simulink model "SrmAmLinearApcZhw3a"  (R2013b)
settings: Solver=ode45  StartTime=0.0  StopTime=10.0  MinStep=5e-5  RelTol=1e-3
InitFcn:
  | theta0=30*2*pi/360;
  | ks=2.44;
  | is=2;
  | lu=0.016;
  | rs=1.5
settings Model: Creator=mamingkai  LastModifiedBy=Think79

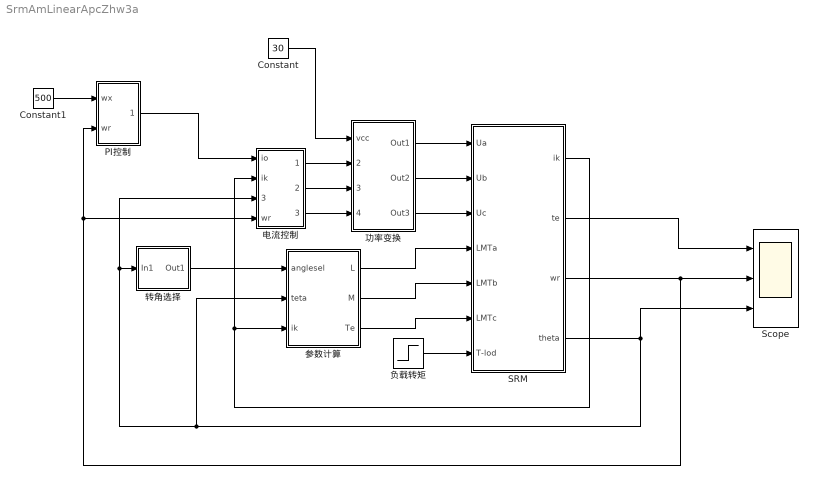
== system SrmAmLinearApcZhw3a ==
  Constant : Constant  Value=30
  Constant1 : Constant  Value=500
  PI控制 : Subsystem
  SRM : Subsystem
  Scope : Scope  NumInputPorts=3
      settings: YMin=-5~-5~-5  YMax=5~5~5
  功率变换 : Subsystem
  参数计算 : Subsystem
  电流控制 : Subsystem
  负载转矩 : Step  SampleTime=0
  转角选择 : Subsystem
  wires:
  Constant1/1 -> PI控制/1(wx)
  电流控制/1(Out1) -> 功率变换/2(PUSEA)
  电流控制/2(Out2) -> 功率变换/3(PUDEB)
  电流控制/3(Out3) -> 功率变换/4(PUSEC)
  PI控制/1(Out1) -> 电流控制/1(io)
  Constant/1 -> 功率变换/1(vcc)
  功率变换/1(Out1) -> SRM/1(Ua)
  功率变换/2(Out2) -> SRM/2(Ub)
  功率变换/3(Out3) -> SRM/3(Uc)
  转角选择/1(Out1) -> 参数计算/1("anglesel ")
  SRM/1(ik) -> 电流控制/2(ik), 参数计算/3(ik)
  SRM/3(wr) -> PI控制/2(wr), 电流控制/4(wr), Scope/2
  SRM/4(theta) -> Scope/3, 参数计算/2(teta), 电流控制/3(teta), 转角选择/1(In1)
  SRM/2(te) -> Scope/1
  参数计算/1(L) -> SRM/4(LMTa)
  参数计算/2(M) -> SRM/5(LMTb)
  参数计算/3(Te) -> SRM/6(LMTc)
  负载转矩/1 -> SRM/7(T-lod)

== system SrmAmLinearApcZhw3a/PI控制 ==
  wx : Inport
  wr : Inport  Port=2
  Gain : Gain
  Gain1 : Gain
  Integrator : Integrator
  Saturation : Saturate
  netsum : Sum  Inputs=2  SaturateOnIntegerOverflow=on  InputSameDT=on  OutDataTypeStr=Inherit: Same as first input
  netsum1 : Sum  Inputs=+-  SaturateOnIntegerOverflow=on  InputSameDT=on  OutDataTypeStr=Inherit: Same as first input
  Out1 : Outport
  wires:
  wx/1 -> netsum1/1
  wr/1 -> netsum1/2
  netsum1/1 -> Gain/1, Gain1/1
  Gain1/1 -> Integrator/1
  Integrator/1 -> netsum/2
  Gain/1 -> netsum/1
  netsum/1 -> Saturation/1
  Saturation/1 -> Out1/1

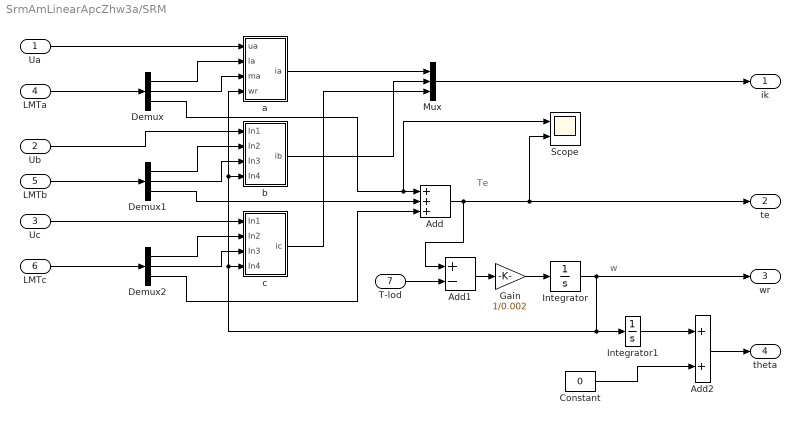
== system SrmAmLinearApcZhw3a/SRM ==
  note: w
  note: Te
  Ua : Inport
  Ub : Inport  Port=2
  Uc : Inport  Port=3
  LMTa : Inport  Port=4
  LMTb : Inport  Port=5
  LMTc : Inport  Port=6
  T-lod : Inport  Port=7
  Add : Sum  Inputs=+++
  Add1 : Sum  Inputs=+-
  Add2 : Sum
  Constant : Constant  Value=0
  Demux : Demux  Outputs=3
  Demux1 : Demux  Outputs=3
  Demux2 : Demux  Outputs=3
  Gain : Gain  Gain=1/0.002
  Integrator : Integrator
  Integrator1 : Integrator
  Mux : Mux  Inputs=3
  Scope : Scope  NumInputPorts=2
      settings: YMin=-5~-5  YMax=5~5
  a : Subsystem
  b : Subsystem
  c : Subsystem
  ik : Outport
  te : Outport  Port=2
  wr : Outport  Port=3
  theta : Outport  Port=4
  wires:
  LMTa/1 -> Demux/1
  Demux/1 -> a/2(la)
  Demux/2 -> a/3(ma)
  Demux/3 -> Scope/1, Add/1
  Ub/1 -> b/1(In1)
  Demux1/1 -> b/2(In2)
  Demux1/2 -> b/3(In3)
  Demux1/3 -> Add/2
  Uc/1 -> c/1(In1)
  LMTc/1 -> Demux2/1
  LMTb/1 -> Demux1/1
  Demux2/1 -> c/2(In2)
  Demux2/2 -> c/3(In3)
  Demux2/3 -> Add/3
  Integrator/1 -> wr/1, c/4(In4), b/4(In4), a/4(wr), Integrator1/1
  a/1(ia) -> Mux/1
  b/1("ib ") -> Mux/2
  c/1(ic) -> Mux/3
  Mux/1 -> ik/1
  Add/1 -> te/1, Scope/2, Add1/1
  T-lod/1 -> Add1/2
  Add1/1 -> Gain/1
  Gain/1 -> Integrator/1
  Add2/1 -> theta/1
  Integrator1/1 -> Add2/1
  Constant/1 -> Add2/2
  Ua/1 -> a/1(ua)

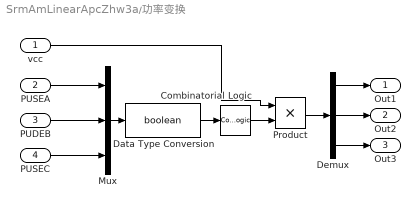
== system SrmAmLinearApcZhw3a/功率变换 ==
  vcc : Inport
  PUSEA : Inport  Port=2
  PUDEB : Inport  Port=3
  PUSEC : Inport  Port=4
  Combinatorial Logic : CombinatorialLogic  TruthTable=[0 0 0 ;0 0 1;0 1 0;0 1 1;1 0 0;1 0 1;1 1 0;1 1 1]
  Data Type Conversion : DataTypeConversion  OutDataTypeStr=boolean
  Demux : Demux  Outputs=3
  Mux : Mux  Inputs=3
  Product : Product
  Out1 : Outport
  Out2 : Outport  Port=2
  Out3 : Outport  Port=3
  wires:
  PUSEA/1 -> Mux/1
  Demux/1 -> Out1/1
  Product/1 -> Demux/1
  Demux/2 -> Out2/1
  Demux/3 -> Out3/1
  PUDEB/1 -> Mux/2
  PUSEC/1 -> Mux/3
  Combinatorial Logic/1 -> Product/2
  vcc/1 -> Product/1
  Mux/1 -> Data Type Conversion/1
  Data Type Conversion/1 -> Combinatorial Logic/1

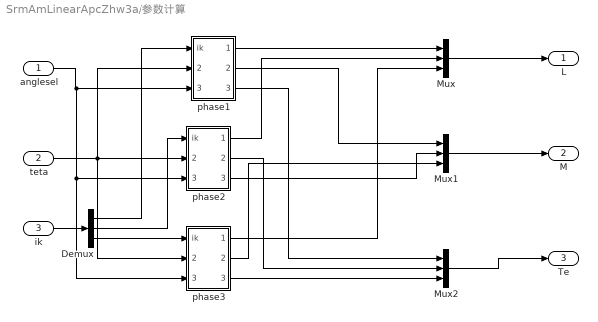
== system SrmAmLinearApcZhw3a/参数计算 ==
  "anglesel " : Inport
  teta : Inport  Port=2
  ik : Inport  Port=3
  Demux : Demux  Outputs=3
  Mux : Mux  Inputs=3
  Mux1 : Mux  Inputs=3
  Mux2 : Mux  Inputs=3
  phase1 : Subsystem
  phase2 : Subsystem
  phase3 : Subsystem
  L : Outport
  M : Outport  Port=2
  Te : Outport  Port=3
  wires:
  teta/1 -> phase3/2(theta), phase2/2(theta), phase1/2(theta)
  Mux/1 -> L/1
  "anglesel "/1 -> phase3/3(angle), phase2/3(angle), phase1/3(angle)
  ik/1 -> Demux/1
  Demux/1 -> phase1/1(ik)
  Demux/2 -> phase2/1(ik)
  Demux/3 -> phase3/1(ik)
  phase1/1(Out1) -> Mux/1
  phase1/2(Out2) -> Mux1/1
  phase1/3(Out3) -> Mux2/1
  phase2/1(Out1) -> Mux/2
  phase2/3(Out3) -> Mux1/2
  phase2/2(Out2) -> Mux2/2
  phase3/1(Out1) -> Mux/3
  phase3/2(Out2) -> Mux1/3
  phase3/3(Out3) -> Mux2/3
  Mux1/1 -> M/1
  Mux2/1 -> Te/1

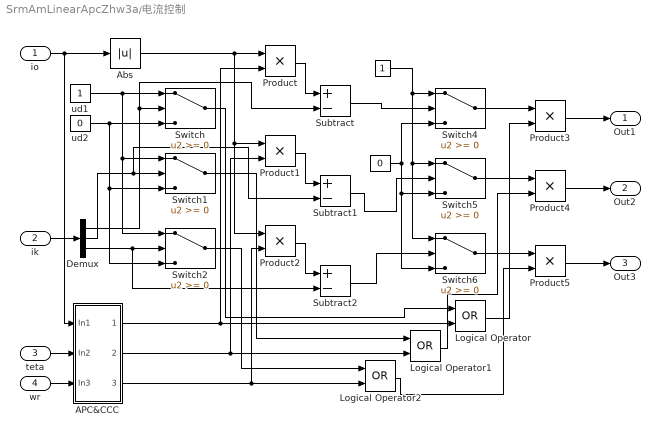
== system SrmAmLinearApcZhw3a/电流控制 ==
  io : Inport
  ik : Inport  Port=2
  teta : Inport  Port=3
  wr : Inport  Port=4
  " " : Constant
  " " : Constant  Value=0
  APC&CCC : Subsystem
  Abs : Abs
  Demux : Demux  Outputs=3
  Logical Operator : Logic  Operator=OR  AllPortsSameDT=off  OutDataTypeStr=boolean
  Logical Operator1 : Logic  Operator=OR  AllPortsSameDT=off  OutDataTypeStr=boolean
  Logical Operator2 : Logic  Operator=OR  AllPortsSameDT=off  OutDataTypeStr=boolean
  Product{,1..5} (6 alike) : Product
  Subtract : Sum  Inputs=+-
  Subtract1 : Sum  Inputs=+-
  Subtract2 : Sum  Inputs=+-
  Switch{,1..2,4..6} (6 alike) : Switch
  ud1 : Constant
  ud2 : Constant  Value=0
  Out1 : Outport
  Out2 : Outport  Port=2
  Out3 : Outport  Port=3
  wires:
  ik/1 -> Demux/1
  io/1 -> APC&CCC/1(In1), Abs/1
  Abs/1 -> Product2/1, Product1/1, Product/1
  ud1/1 -> Switch2/1, Switch1/1, Switch/1
  ud2/1 -> Switch2/3, Switch1/3, Switch/3
  teta/1 -> APC&CCC/2(In2)
  Demux/1 -> Subtract/2, Switch/2
  Demux/3 -> Subtract2/2, Switch2/2
  Demux/2 -> Subtract1/2, Switch1/2
  APC&CCC/1(Out1) -> Product/2, Logical Operator/2
  APC&CCC/2(Out2) -> Product1/2, Logical Operator1/2
  APC&CCC/3(Out3) -> Product2/2, Logical Operator2/2
  Switch/1 -> Logical Operator/1
  Switch1/1 -> Logical Operator1/1
  Switch2/1 -> Logical Operator2/1
  Product/1 -> Subtract/1
  Product1/1 -> Subtract1/1
  Product2/1 -> Subtract2/1
  " "/1 -> Switch6/1, Switch5/1, Switch4/1
  " "/1 -> Switch6/3, Switch5/3, Switch4/3
  wr/1 -> APC&CCC/3(In3)
  Logical Operator/1 -> Product3/2
  Logical Operator1/1 -> Product4/2
  Logical Operator2/1 -> Product5/2
  Switch6/1 -> Product5/1
  Switch5/1 -> Product4/1
  Switch4/1 -> Product3/1
  Product3/1 -> Out1/1
  Product4/1 -> Out2/1
  Product5/1 -> Out3/1
  Subtract1/1 -> Switch5/2
  Subtract/1 -> Switch4/2
  Subtract2/1 -> Switch6/2

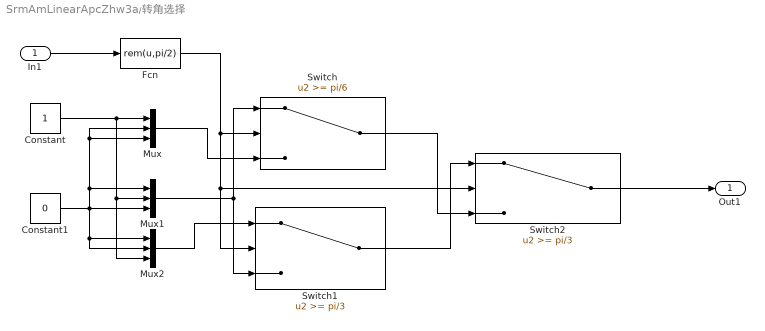
== system SrmAmLinearApcZhw3a/转角选择 ==
  In1 : Inport
  Constant : Constant
  Constant1 : Constant  Value=0
  Fcn : Fcn  Expr=rem(u,pi/2)
  Mux : Mux  Inputs=3
  Mux1 : Mux  Inputs=3
  Mux2 : Mux  Inputs=3
  Switch : Switch  Threshold=pi/6
  Switch1 : Switch  Threshold=pi/3
  Switch2 : Switch  Threshold=pi/3
  Out1 : Outport
  wires:
  In1/1 -> Fcn/1
  Constant/1 -> Mux2/3, Mux1/2, Mux/1
  Mux/1 -> Switch/3
  Constant1/1 -> Mux/3, Mux/2, Mux1/1, Mux2/2, Mux2/1, Mux1/3
  Mux1/1 -> Switch1/3, Switch/1
  Mux2/1 -> Switch1/1
  Fcn/1 -> Switch2/2, Switch1/2, Switch/2
  Switch/1 -> Switch2/3
  Switch1/1 -> Switch2/1
  Switch2/1 -> Out1/1

== system SrmAmLinearApcZhw3a/SRM/a ==
  ua : Inport
  la : Inport  Port=2
  ma : Inport  Port=3
  wr : Inport  Port=4
  Add : Sum  Inputs=+--
  Fcn : Fcn  Expr=1/u
  Gain : Gain  Gain=rs
  Integrator : Integrator
  Product : Product
  Product1 : Product
  ia : Outport
  wires:
  wr/1 -> Product/2
  Integrator/1 -> Gain/1, ia/1
  ma/1 -> Product/1
  la/1 -> Fcn/1
  ua/1 -> Add/1
  Gain/1 -> Add/2
  Product/1 -> Add/3
  Add/1 -> Product1/1
  Fcn/1 -> Product1/2
  Product1/1 -> Integrator/1

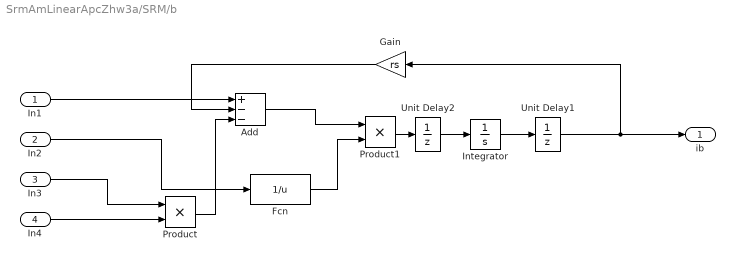
== system SrmAmLinearApcZhw3a/SRM/b ==
  In1 : Inport
  In2 : Inport  Port=2
  In3 : Inport  Port=3
  In4 : Inport  Port=4
  Add : Sum  Inputs=+--
  Fcn : Fcn  Expr=1/u
  Gain : Gain  Gain=rs
  Integrator : Integrator
  Product : Product
  Product1 : Product
  Unit Delay1 : UnitDelay  SampleTime=-1
  Unit Delay2 : UnitDelay  SampleTime=-1
  "ib " : Outport
  wires:
  In4/1 -> Product/2
  Integrator/1 -> Unit Delay1/1
  In3/1 -> Product/1
  In2/1 -> Fcn/1
  In1/1 -> Add/1
  Gain/1 -> Add/2
  Product/1 -> Add/3
  Add/1 -> Product1/1
  Fcn/1 -> Product1/2
  Product1/1 -> Unit Delay2/1
  Unit Delay2/1 -> Integrator/1
  Unit Delay1/1 -> Gain/1, "ib "/1

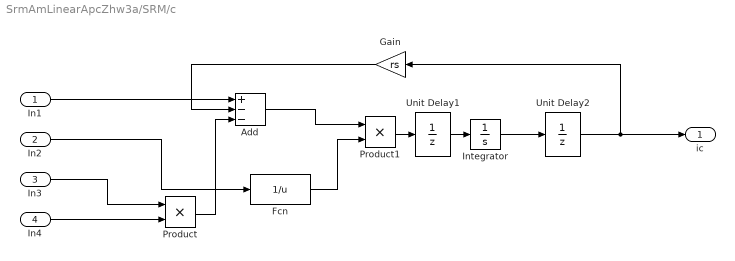
== system SrmAmLinearApcZhw3a/SRM/c ==
  In1 : Inport
  In2 : Inport  Port=2
  In3 : Inport  Port=3
  In4 : Inport  Port=4
  Add : Sum  Inputs=+--
  Fcn : Fcn  Expr=1/u
  Gain : Gain  Gain=rs
  Integrator : Integrator  InitialCondition=1e-5
  Product : Product
  Product1 : Product
  Unit Delay1 : UnitDelay  SampleTime=-1
  Unit Delay2 : UnitDelay  SampleTime=-1
  ic : Outport
  wires:
  In4/1 -> Product/2
  Integrator/1 -> Unit Delay2/1
  In3/1 -> Product/1
  In2/1 -> Fcn/1
  In1/1 -> Add/1
  Gain/1 -> Add/2
  Product/1 -> Add/3
  Add/1 -> Product1/1
  Fcn/1 -> Product1/2
  Product1/1 -> Unit Delay1/1
  Unit Delay2/1 -> Gain/1, ic/1
  Unit Delay1/1 -> Integrator/1

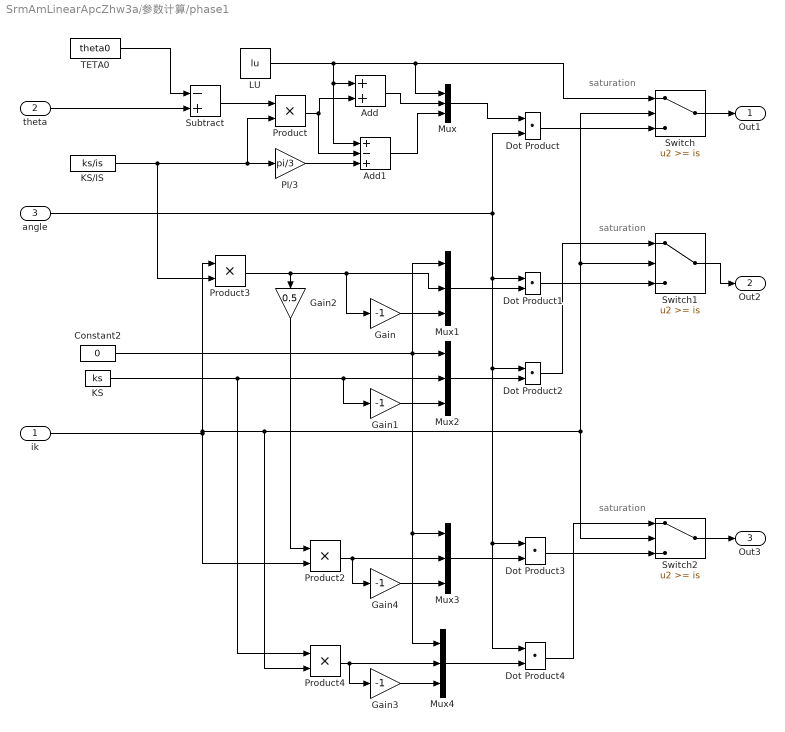
== system SrmAmLinearApcZhw3a/参数计算/phase1 ==
  note: saturation
  note: saturation
  note: saturation
  ik : Inport
  theta : Inport  Port=2
  angle : Inport  Port=3
  Add : Sum
  Add1 : Sum  Inputs=+-+
  Constant2 : Constant  Value=0
  Dot Product{,1..4} (5 alike) : DotProduct  InputSameDT=on  OutDataTypeStr=Inherit: Inherit via internal rule
  Gain{,1,3..4} (4 alike) : Gain  Gain=-1
  Gain2 : Gain  Gain=0.5
  KS : Constant  Value=ks
  KS/IS : Constant  Value=ks/is
  LU : Constant  Value=lu
  Mux{,1..4} (5 alike) : Mux  Inputs=3
  PI/3 : Gain  Gain=pi/3
  Product{,2..4} (4 alike) : Product
  Subtract : Sum  Inputs=-+
  Switch : Switch  Threshold=is
  Switch1 : Switch  Threshold=is
  Switch2 : Switch  Threshold=is
  TETA0 : Constant  Value=theta0
  Out1 : Outport
  Out2 : Outport  Port=2
  Out3 : Outport  Port=3
  wires:
  Switch/1 -> Out1/1
  theta/1 -> Subtract/2
  TETA0/1 -> Subtract/1
  Subtract/1 -> Product/1
  KS/IS/1 -> Product3/2, PI/3/1, Product/2
  LU/1 -> Switch/1, Mux/1, Add1/1, Add/1
  Product/1 -> Add1/2, Add/2
  PI/3/1 -> Add1/3
  Add/1 -> Mux/2
  Add1/1 -> Mux/3
  Mux/1 -> Dot Product/1
  Dot Product/1 -> Switch/3
  ik/1 -> Product3/1, Product4/2, Switch/2, Switch1/2, Switch2/2, Product2/2
  angle/1 -> Dot Product4/1, Dot Product3/1, Dot Product2/1, Dot Product1/1, Dot Product/2
  Mux4/1 -> Dot Product4/2
  Constant2/1 -> Mux1/1, Mux4/1, Mux3/1, Mux2/1
  Mux3/1 -> Dot Product3/2
  Mux2/1 -> Dot Product2/2
  Mux1/1 -> Dot Product1/2
  KS/1 -> Product4/1, Gain1/1, Mux2/2
  Product3/1 -> Gain/1, Mux1/2, Gain2/1
  Gain/1 -> Mux1/3
  Gain2/1 -> Product2/1
  Product4/1 -> Mux4/2, Gain3/1
  Gain3/1 -> Mux4/3
  Dot Product4/1 -> Switch2/1
  Dot Product3/1 -> Switch2/3
  Dot Product2/1 -> Switch1/1
  Dot Product1/1 -> Switch1/3
  Switch1/1 -> Out2/1
  Switch2/1 -> Out3/1
  Product2/1 -> Gain4/1, Mux3/2
  Gain4/1 -> Mux3/3
  Gain1/1 -> Mux2/3

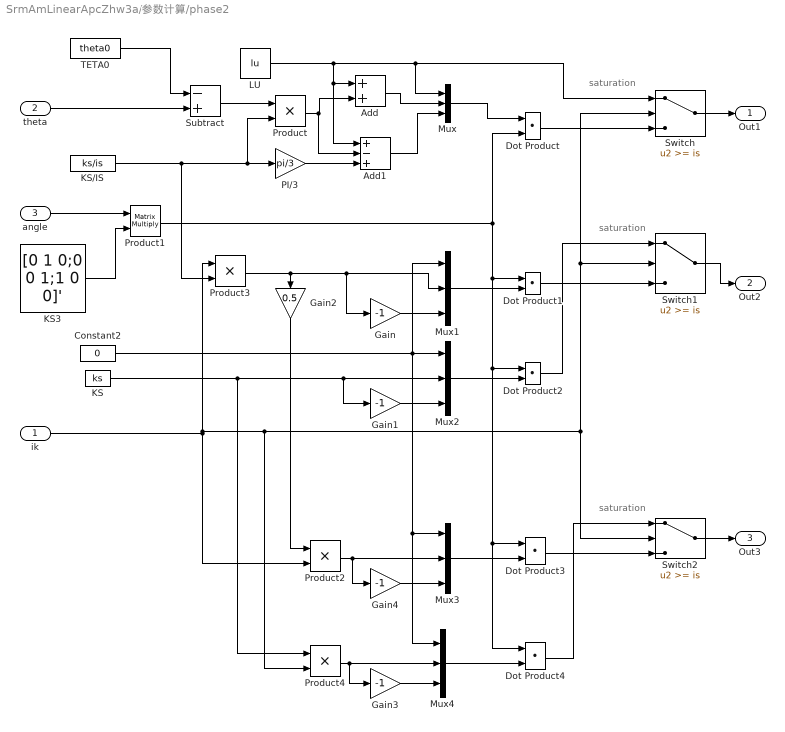
== system SrmAmLinearApcZhw3a/参数计算/phase2 ==
  note: saturation
  note: saturation
  note: saturation
  ik : Inport
  theta : Inport  Port=2
  angle : Inport  Port=3
  Add : Sum
  Add1 : Sum  Inputs=+-+
  Constant2 : Constant  Value=0
  Dot Product{,1..4} (5 alike) : DotProduct  InputSameDT=on  OutDataTypeStr=Inherit: Inherit via internal rule
  Gain{,1,3..4} (4 alike) : Gain  Gain=-1
  Gain2 : Gain  Gain=0.5
  KS : Constant  Value=ks
  KS/IS : Constant  Value=ks/is
  KS3 : Constant  Value="[0 1 0;0  0 1;1 0 0]'"  VectorParams1D=off
  LU : Constant  Value=lu
  Mux{,1..4} (5 alike) : Mux  Inputs=3
  PI/3 : Gain  Gain=pi/3
  Product{,2..4} (4 alike) : Product
  Product1 : Product  Multiplication=Matrix(*)
  Subtract : Sum  Inputs=-+
  Switch : Switch  Threshold=is
  Switch1 : Switch  Threshold=is
  Switch2 : Switch  Threshold=is
  TETA0 : Constant  Value=theta0
  Out1 : Outport
  Out2 : Outport  Port=2
  Out3 : Outport  Port=3
  wires:
  Switch/1 -> Out1/1
  theta/1 -> Subtract/2
  TETA0/1 -> Subtract/1
  Subtract/1 -> Product/1
  KS/IS/1 -> Product3/2, PI/3/1, Product/2
  LU/1 -> Switch/1, Mux/1, Add1/1, Add/1
  Product/1 -> Add1/2, Add/2
  PI/3/1 -> Add1/3
  Add/1 -> Mux/2
  Add1/1 -> Mux/3
  Mux/1 -> Dot Product/1
  Dot Product/1 -> Switch/3
  ik/1 -> Product3/1, Product4/2, Switch/2, Switch1/2, Switch2/2, Product2/2
  Product1/1 -> Dot Product/2, Dot Product4/1, Dot Product3/1, Dot Product2/1, Dot Product1/1
  Mux4/1 -> Dot Product4/2
  Constant2/1 -> Mux1/1, Mux4/1, Mux3/1, Mux2/1
  Mux3/1 -> Dot Product3/2
  Mux2/1 -> Dot Product2/2
  Mux1/1 -> Dot Product1/2
  KS/1 -> Product4/1, Gain1/1, Mux2/2
  Product3/1 -> Gain/1, Mux1/2, Gain2/1
  Gain/1 -> Mux1/3
  Gain2/1 -> Product2/1
  Product4/1 -> Mux4/2, Gain3/1
  Gain3/1 -> Mux4/3
  Dot Product4/1 -> Switch2/1
  Dot Product3/1 -> Switch2/3
  Dot Product2/1 -> Switch1/1
  Dot Product1/1 -> Switch1/3
  Switch1/1 -> Out2/1
  Switch2/1 -> Out3/1
  Product2/1 -> Gain4/1, Mux3/2
  Gain4/1 -> Mux3/3
  Gain1/1 -> Mux2/3
  KS3/1 -> Product1/2
  angle/1 -> Product1/1

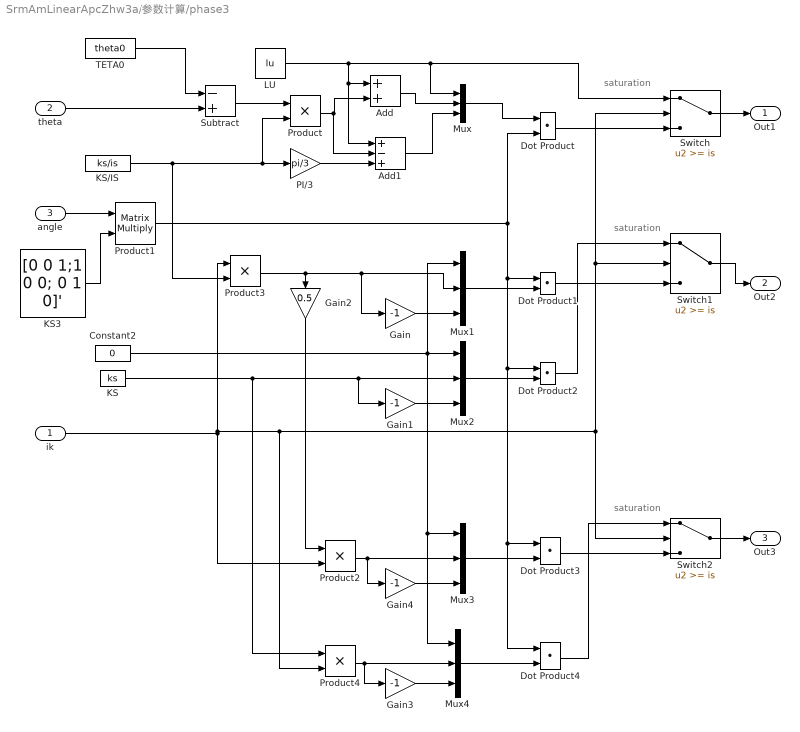
== system SrmAmLinearApcZhw3a/参数计算/phase3 ==
  note: saturation
  note: saturation
  note: saturation
  ik : Inport
  theta : Inport  Port=2
  angle : Inport  Port=3
  Add : Sum
  Add1 : Sum  Inputs=+-+
  Constant2 : Constant  Value=0
  Dot Product{,1..4} (5 alike) : DotProduct  InputSameDT=on  OutDataTypeStr=Inherit: Inherit via internal rule
  Gain{,1,3..4} (4 alike) : Gain  Gain=-1
  Gain2 : Gain  Gain=0.5
  KS : Constant  Value=ks
  KS/IS : Constant  Value=ks/is
  KS3 : Constant  Value="[0 0 1;1 0  0; 0 1 0]'"  VectorParams1D=off
  LU : Constant  Value=lu
  Mux{,1..4} (5 alike) : Mux  Inputs=3
  PI/3 : Gain  Gain=pi/3
  Product{,2..4} (4 alike) : Product
  Product1 : Product  Multiplication=Matrix(*)
  Subtract : Sum  Inputs=-+
  Switch : Switch  Threshold=is
  Switch1 : Switch  Threshold=is
  Switch2 : Switch  Threshold=is
  TETA0 : Constant  Value=theta0
  Out1 : Outport
  Out2 : Outport  Port=2
  Out3 : Outport  Port=3
  wires:
  Switch/1 -> Out1/1
  theta/1 -> Subtract/2
  TETA0/1 -> Subtract/1
  Subtract/1 -> Product/1
  KS/IS/1 -> Product3/2, PI/3/1, Product/2
  LU/1 -> Switch/1, Mux/1, Add1/1, Add/1
  Product/1 -> Add1/2, Add/2
  PI/3/1 -> Add1/3
  Add/1 -> Mux/2
  Add1/1 -> Mux/3
  Mux/1 -> Dot Product/1
  Dot Product/1 -> Switch/3
  ik/1 -> Product3/1, Product4/2, Switch/2, Switch1/2, Switch2/2, Product2/2
  Product1/1 -> Dot Product4/1, Dot Product3/1, Dot Product2/1, Dot Product1/1, Dot Product/2
  Mux4/1 -> Dot Product4/2
  Constant2/1 -> Mux1/1, Mux4/1, Mux3/1, Mux2/1
  Mux3/1 -> Dot Product3/2
  Mux2/1 -> Dot Product2/2
  Mux1/1 -> Dot Product1/2
  KS/1 -> Product4/1, Gain1/1, Mux2/2
  Product3/1 -> Gain/1, Mux1/2, Gain2/1
  Gain/1 -> Mux1/3
  Gain2/1 -> Product2/1
  Product4/1 -> Mux4/2, Gain3/1
  Gain3/1 -> Mux4/3
  Dot Product4/1 -> Switch2/1
  Dot Product3/1 -> Switch2/3
  Dot Product2/1 -> Switch1/1
  Dot Product1/1 -> Switch1/3
  Switch1/1 -> Out2/1
  Switch2/1 -> Out3/1
  Product2/1 -> Gain4/1, Mux3/2
  Gain4/1 -> Mux3/3
  Gain1/1 -> Mux2/3
  angle/1 -> Product1/1
  KS3/1 -> Product1/2

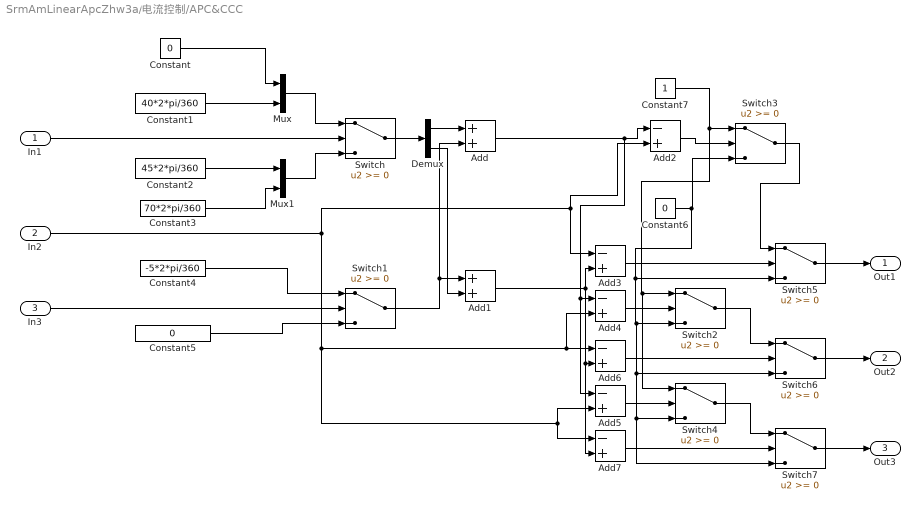
== system SrmAmLinearApcZhw3a/电流控制/APC&CCC ==
  In1 : Inport
  In2 : Inport  Port=2
  In3 : Inport  Port=3
  Add : Sum
  Add1 : Sum
  Add{2..7} (6 alike) : Sum  Inputs=-+
  Constant : Constant  Value=0
  Constant1 : Constant  Value=40*2*pi/360
  Constant2 : Constant  Value=45*2*pi/360
  Constant3 : Constant  Value=70*2*pi/360
  Constant4 : Constant  Value=-5*2*pi/360
  Constant5 : Constant  Value=0
  Constant6 : Constant  Value=0
  Constant7 : Constant
  Demux : Demux  Outputs=2
  Mux : Mux  Inputs=2
  Mux1 : Mux  Inputs=2
  Switch{,1..7} (8 alike) : Switch
  Out1 : Outport
  Out2 : Outport  Port=2
  Out3 : Outport  Port=3
  wires:
  Switch5/1 -> Out1/1
  In3/1 -> Switch1/2
  In1/1 -> Switch/2
  Mux/1 -> Switch/1
  Constant4/1 -> Switch1/1
  Constant5/1 -> Switch1/3
  Constant/1 -> Mux/1
  Constant1/1 -> Mux/2
  Constant2/1 -> Mux1/1
  Constant3/1 -> Mux1/2
  Mux1/1 -> Switch/3
  Switch/1 -> Demux/1
  Demux/1 -> Add/1
  Demux/2 -> Add1/2
  Switch1/1 -> Add1/1, Add/2
  Add1/1 -> Add3/2, Add6/2, Add7/2
  Add/1 -> Add5/1, Add4/1, Add2/1
  In2/1 -> Add2/2, Add3/1, Add7/1, Add5/2, Add6/1, Add4/2
  Add3/1 -> Switch5/2
  Add4/1 -> Switch2/2
  Add6/1 -> Switch6/2
  Add5/1 -> Switch4/2
  Add7/1 -> Switch7/2
  Constant7/1 -> Switch4/1, Switch2/1, Switch3/1
  Constant6/1 -> Switch6/3, Switch7/3, Switch4/3, Switch2/3, Switch5/3, Switch3/3
  Switch3/1 -> Switch5/1
  Switch2/1 -> Switch6/1
  Switch4/1 -> Switch7/1
  Switch6/1 -> Out2/1
  Switch7/1 -> Out3/1
  Add2/1 -> Switch3/2
